simulink model "FixedWing_Dynamic_Model_SIL_simulink_PX4"  (R2023a)
settings: Solver=ode4  StartTime=0.0  StopTime=130  FixedStep=0.004  RelTol=1e-3
model workspace (MAT data in the model file):
  sample_time = 0.004
values from neighbouring files (symbols this model uses):
  env = struct    [InitEnvironment.m]
  frecuency = 0.012    [PX4_var_controllers.m]
  g = 9.81    [PX4_var_controllers.m]
  home_alt = 171    [InitSimulinkPlantVars.m]    (also in PX4_var_controllers.m)
  home_lat = 39.49738807491014    (= 39.4973880749)    [InitSimulinkPlantVars.m]    (also in PX4_var_controllers.m)
  home_lon = -0.6268122488722822    (= -0.626812248872)    [InitSimulinkPlantVars.m]    (also in PX4_var_controllers.m)
  mission = [wp]    [PX4_var_controllers.m]
  nwap = 9    [PX4_var_controllers.m]
  pitch_D = 0    [PX4_var_controllers.m]
  pitch_ff = 0.4    [PX4_var_controllers.m]
  pitch_I = 0.05    [PX4_var_controllers.m]
  pitch_P = 0.05    [PX4_var_controllers.m]
  poswp = [poswp1;poswp2;poswp3;poswp4;poswp5;poswp6;poswp7;poswp8;poswp9]    [PX4_var_controllers.m]
  roll_D = 0    [PX4_var_controllers.m]
  roll_ff = 0.4    [PX4_var_controllers.m]
  roll_I = 0.13    [PX4_var_controllers.m]
  roll_P = 0.085    [PX4_var_controllers.m]
  tc_pitch = 0.4    [PX4_var_controllers.m]
  tc_roll = 0.45    [PX4_var_controllers.m]
  uavData = struct    [InitFixedWingParam.m]
  V_cruise = [15,15,15,20,25,25,20,15,15]    [PX4_var_controllers.m]
  yaw_D = 0    [PX4_var_controllers.m]
  yaw_ff = 0.3    [PX4_var_controllers.m]
  yaw_I = 0.1    [PX4_var_controllers.m]
  yaw_P = 0.05    [PX4_var_controllers.m]
undefined symbols (not defined in the file or in its folder): DiscIntNeverNeededParam, Earth, LC, TEBCL, TECL, TECS, WGS84
libraries: aerolibactuator x5, aerolibasang x4, slpidlib x3, uavalgslib x2, aerolibatmos2 x2, shared6dof x1, aerolibtransform2 x1, aerolibconvert2 x1, simulink_extras x1
(part 2 of 3)

== system FixedWing_Dynamic_Model_SIL_simulink_PX4/Dynamics/Fixed-wing UAV Dynamics/Force and Moment Calculation ==
  note: M. Lizarraga. Design, Implementation and Flight Verification of a Versatile and Rapidly Reconfigurable UAV GNC Research Platform. PhD Dissertation, UC, Santa Cruz, Santa Cruz, CA, USA, 2009
  DCMbe : Inport
  Ve : Inport  Port=2
  Xe : Inport  Port=3
  pqr_b : Inport  Port=4
  rpy : Inport  Port=5
  Inputs : Inport  Port=6
  Actuator Model : Subsystem
  Add : Sum  Inputs=4
  Add1 : Sum  Inputs=2
  Aerodynamic Forces and Moments : Subsystem
  Bus Selector : BusSelector  OutputSignals=airspeed
  Constant : Constant  Value=[0 0 0]
  Gravity : Subsystem
  Ground Model : Subsystem
  Motor Model : Subsystem
  Terminator : Terminator
  F_xyz : Outport
  M_xyz : Outport  Port=2
  Airspeed : Outport  Port=3
  wires:
  Add/1 -> F_xyz/1
  DCMbe/1 -> Aerodynamic Forces and Moments/4(DCM_be), Ground Model/1(DCMbe), Gravity/1(DCM_be)
  pqr_b/1 -> Ground Model/5(pqr_b), Aerodynamic Forces and Moments/6(pqr_b)
  Actuator Model/1(ctrlSurfaces) -> Aerodynamic Forces and Moments/1(CtrlSurfaces), Motor Model/1(Ctrl Surfaces)
  Aerodynamic Forces and Moments/1(AirData) -> Bus Selector/1, Motor Model/2(Air Data)
  Ground Model/1(Fb_contact) -> Add/4
  Gravity/1(Fb_g) -> Add/3
  Motor Model/1(Fb_motor) -> Add/1
  Ve/1 -> Aerodynamic Forces and Moments/3(Ve), Ground Model/3(Ve)
  Ground Model/3(Crash_flag) -> Terminator/1
  Aerodynamic Forces and Moments/2(Fb_aero) -> Add/2
  Aerodynamic Forces and Moments/3(Mb_aero) -> Add1/1
  Xe/1 -> Aerodynamic Forces and Moments/5(Xe), Ground Model/2(Xe)
  Constant/1 -> Aerodynamic Forces and Moments/2(Wind_e)
  Inputs/1 -> Actuator Model/1(CtrlCmds)
  Bus Selector/1 -> Airspeed/1  "<airspeed>"
  rpy/1 -> Ground Model/4(rpy)
  Add1/1 -> M_xyz/1
  Ground Model/2(Mb_contact) -> Add1/2

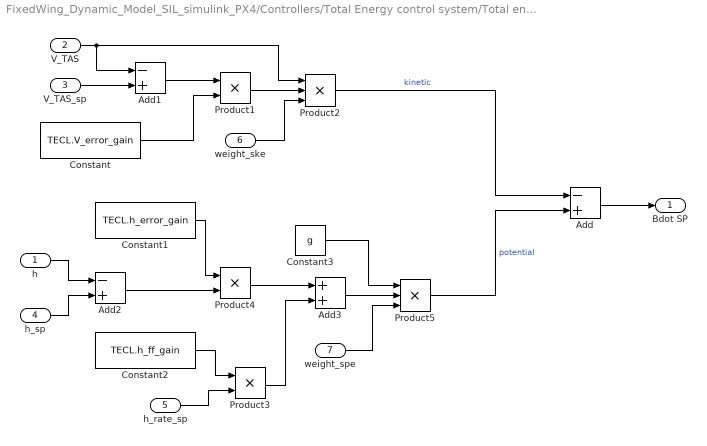
== system FixedWing_Dynamic_Model_SIL_simulink_PX4/Controllers/Total Energy control system/Total energy balance control loop/ B SP dot ==
  h : Inport  SampleTime=frecuency
  V_TAS : Inport  Port=2  SampleTime=frecuency
  V_TAS_sp : Inport  Port=3  SampleTime=frecuency
  h_sp : Inport  Port=4  SampleTime=frecuency
  h_rate_sp : Inport  Port=5  SampleTime=frecuency
  weight_ske : Inport  Port=6  SampleTime=frecuency
  weight_spe : Inport  Port=7  SampleTime=frecuency
  Add : Sum  Inputs=-+
  Add1 : Sum  Inputs=-+
  Add2 : Sum  Inputs=-+
  Add3 : Sum
  Constant : Constant  Value=TECL.V_error_gain  SampleTime=frecuency
  Constant1 : Constant  Value=TECL.h_error_gain  SampleTime=frecuency
  Constant2 : Constant  Value=TECL.h_ff_gain  SampleTime=frecuency
  Constant3 : Constant  Value=g  SampleTime=frecuency
  Product1 : Product
  Product2 : Product  Inputs=3
  Product3 : Product
  Product4 : Product
  Product5 : Product  Inputs=3
  Bdot SP : Outport  SampleTime=frecuency
  wires:
  V_TAS_sp/1 -> Add1/2
  Product1/1 -> Product2/2
  Product2/1 -> Add/1  "kinetic"
  h_sp/1 -> Add2/2
  h/1 -> Add2/1
  Add2/1 -> Product4/2
  Constant1/1 -> Product4/1
  Product4/1 -> Add3/1
  Constant2/1 -> Product3/1
  Product3/1 -> Add3/2
  Add3/1 -> Product5/2
  Constant3/1 -> Product5/1
  Product5/1 -> Add/2  "potential"
  Add/1 -> Bdot SP/1
  h_rate_sp/1 -> Product3/2
  weight_ske/1 -> Product2/3
  weight_spe/1 -> Product5/3
  V_TAS/1 -> Add1/1, Product2/1
  Add1/1 -> Product1/1
  Constant/1 -> Product1/2

== system FixedWing_Dynamic_Model_SIL_simulink_PX4/Controllers/Total Energy control system/Total energy balance control loop/Bdot ==
  V_TAS : Inport  SampleTime=frecuency
  V_rate : Inport  Port=2  SampleTime=frecuency
  h_rate : Inport  Port=3  SampleTime=frecuency
  weight_ske : Inport  Port=4  SampleTime=frecuency
  weight_spe : Inport  Port=5  SampleTime=frecuency
  Add : Sum  Inputs=-+
  Constant : Constant  Value=g  SampleTime=frecuency
  Product : Product  Inputs=3
  Product1 : Product  Inputs=3
  Bdot : Outport  SampleTime=frecuency
  wires:
  V_rate/1 -> Product/2
  Constant/1 -> Product1/3
  h_rate/1 -> Product1/2
  Product/1 -> Add/1  "kinetic"
  Product1/1 -> Add/2  "potential"
  Add/1 -> Bdot/1
  weight_ske/1 -> Product/3
  weight_spe/1 -> Product1/1
  V_TAS/1 -> Product/1

== system FixedWing_Dynamic_Model_SIL_simulink_PX4/Controllers/Total Energy control system/Total energy balance control loop/pitchdotsp - pitchFF ==
  Bdot SP : Inport  SampleTime=frecuency
  Gain : Gain  Gain=TEBCL.rate_ff
  pitch_FF : Outport  SampleTime=frecuency
  wires:
  Bdot SP/1 -> Gain/1
  Gain/1 -> pitch_FF/1

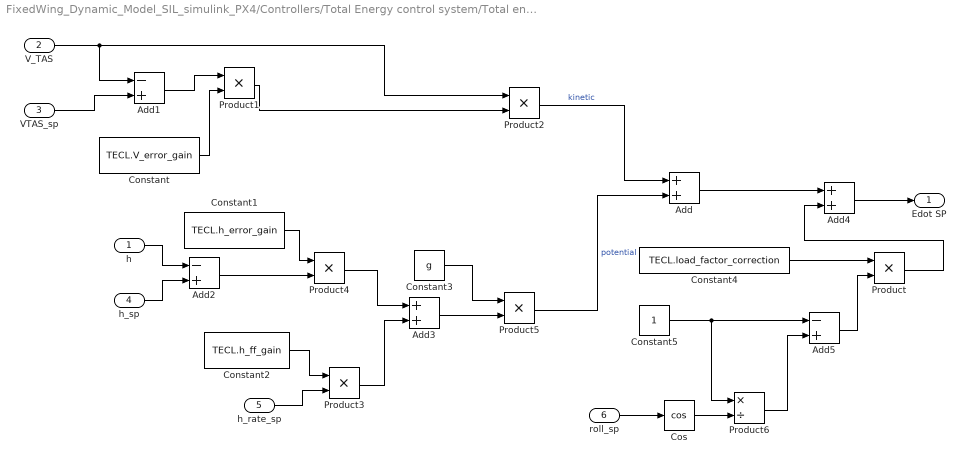
== system FixedWing_Dynamic_Model_SIL_simulink_PX4/Controllers/Total Energy control system/Total energy control loop/E SP dot ==
  h : Inport  SampleTime=frecuency
  V_TAS : Inport  Port=2  SampleTime=frecuency
  VTAS_sp : Inport  Port=3  SampleTime=frecuency
  h_sp : Inport  Port=4  SampleTime=frecuency
  h_rate_sp : Inport  Port=5  SampleTime=frecuency
  roll_sp : Inport  Port=6  SampleTime=frecuency
  Add : Sum
  Add1 : Sum  Inputs=-+
  Add2 : Sum  Inputs=-+
  Add3 : Sum
  Add4 : Sum
  Add5 : Sum  Inputs=-+
  Constant : Constant  Value=TECL.V_error_gain  SampleTime=frecuency
  Constant1 : Constant  Value=TECL.h_error_gain  SampleTime=frecuency
  Constant2 : Constant  Value=TECL.h_ff_gain  SampleTime=frecuency
  Constant3 : Constant  Value=g
  Constant4 : Constant  Value=TECL.load_factor_correction  SampleTime=frecuency
  Constant5 : Constant
  Cos : Trigonometry  Operator=cos
  Product{,1..5} (6 alike) : Product
  Product6 : Product  Inputs=*/
  Edot SP : Outport  SampleTime=frecuency
  wires:
  VTAS_sp/1 -> Add1/2
  Product2/1 -> Add/1  "kinetic"
  h_sp/1 -> Add2/2
  h/1 -> Add2/1
  Add2/1 -> Product4/2
  Constant1/1 -> Product4/1
  Product4/1 -> Add3/1
  Constant2/1 -> Product3/1
  Product3/1 -> Add3/2
  Add3/1 -> Product5/2
  Constant3/1 -> Product5/1
  Product5/1 -> Add/2  "potential"
  h_rate_sp/1 -> Product3/2
  Add/1 -> Add4/1
  Add4/1 -> Edot SP/1
  Constant4/1 -> Product/1
  Product/1 -> Add4/2
  Constant5/1 -> Add5/1, Product6/1
  Add5/1 -> Product/2
  roll_sp/1 -> Cos/1
  Cos/1 -> Product6/2
  Product6/1 -> Add5/2
  Constant/1 -> Product1/2
  Add1/1 -> Product1/1
  Product1/1 -> Product2/2
  V_TAS/1 -> Product2/1, Add1/1

== system FixedWing_Dynamic_Model_SIL_simulink_PX4/Controllers/Total Energy control system/Total energy control loop/Edot ==
  V_TAS : Inport  SampleTime=frecuency
  V_rate : Inport  Port=2  SampleTime=frecuency
  h_rate : Inport  Port=3  SampleTime=frecuency
  Add : Sum
  Constant : Constant  Value=g  SampleTime=frecuency
  Product : Product
  Product1 : Product
  Edot : Outport  SampleTime=frecuency
  wires:
  V_TAS/1 -> Product/1
  V_rate/1 -> Product/2
  Constant/1 -> Product1/2
  h_rate/1 -> Product1/1
  Product/1 -> Add/1  "kinetic"
  Product1/1 -> Add/2  "potential"
  Add/1 -> Edot/1

== system FixedWing_Dynamic_Model_SIL_simulink_PX4/Controllers/Total Energy control system/Total energy control loop/Subsystem ==
  ratio_undersped : Inport  SampleTime=frecuency
  T_sp : Inport  Port=2  SampleTime=frecuency
  Tmax : Inport  Port=3  SampleTime=frecuency
  Add : Sum  Inputs=+-
  Add1 : Sum
  Constant : Constant  SampleTime=frecuency
  Product : Product
  Product1 : Product
  throttle_setpoint : Outport  SampleTime=frecuency
  wires:
  ratio_undersped/1 -> Product/1, Add/2
  Tmax/1 -> Product/2
  Constant/1 -> Add/1
  T_sp/1 -> Product1/1
  Add/1 -> Product1/2
  Product1/1 -> Add1/1
  Product/1 -> Add1/2
  Add1/1 -> throttle_setpoint/1

== system FixedWing_Dynamic_Model_SIL_simulink_PX4/Controllers/Total Energy control system/Total energy control loop/Subsystem1 ==
  throttle_integ_input : Inport  SampleTime=frecuency
  ste_rate_to_throttle : Inport  Port=2  SampleTime=frecuency
  ratio_undersped : Inport  Port=3  SampleTime=frecuency
  Add : Sum  Inputs=-+
  Constant : Constant  SampleTime=frecuency
  Product : Product  Inputs=3
  throttle_integ : Outport  SampleTime=frecuency
  wires:
  ratio_undersped/1 -> Add/1
  Constant/1 -> Add/2
  throttle_integ_input/1 -> Product/1
  ste_rate_to_throttle/1 -> Product/2
  Add/1 -> Product/3
  Product/1 -> throttle_integ/1

== system FixedWing_Dynamic_Model_SIL_simulink_PX4/Dynamics/Fixed-wing UAV Dynamics/Force and Moment Calculation/Actuator Model ==
  note: Simple Actuator Model
  note: MAIN1 : aileron
      | MAIN2 : elevator
      | MAIN3 : rudder
      | MAIN4 : throttle
  CtrlCmds : Inport
  Bus Creator1 : BusCreator  Inputs=5
  Constant : Constant  Value=0*pi/180
  Demux : Demux
  Linear Second Order Actuators : aerolibactuator/Linear Second-Order Actuator  wn_fin=35  z_fin=0.75  fin_act_0=0  fin_act_vel=0
      settings: AttributesFormatString=|
      | Nat Freq => %<wn_fin>
      | Damping => %<z_fin>
  Linear Second-Order Actuator{1..4} (4 alike) : aerolibactuator/Linear Second-Order Actuator  wn_fin=35  z_fin=0.75  fin_act_0=0  fin_act_vel=0
  Signal Specification{,1..3} (4 alike) : SignalSpecification  Unit=rad
  Signal Specification4 : SignalSpecification  Unit=%
  uavData.cntrl.aileronGain : Gain  Gain=uavData.cntrl.aieleronGain
  uavData.cntrl.elevatorGain : Gain  Gain=uavData.cntrl.elevatorGain
  uavData.cntrl.rudderGain : Gain  Gain=uavData.cntrl.rudderGain
  uavData.cntrl.throttleGain : Gain  Gain=uavData.cntrl.throttleGain
  ctrlSurfaces : Outport  VectorParamsAs1DForOutWhenUnconnected=off
  wires:
  uavData.cntrl.elevatorGain/1 -> Linear Second-Order Actuator4/1
  uavData.cntrl.aileronGain/1 -> Linear Second-Order Actuator3/1
  uavData.cntrl.rudderGain/1 -> Linear Second-Order Actuator2/1
  Constant/1 -> Linear Second-Order Actuator1/1
  Bus Creator1/1 -> ctrlSurfaces/1
  Linear Second-Order Actuator4/1 -> Signal Specification1/1  "dE"
  Linear Second-Order Actuator3/1 -> Signal Specification/1  "dA"
  Linear Second-Order Actuator2/1 -> Signal Specification2/1  "dR"
  Linear Second-Order Actuator1/1 -> Signal Specification3/1  "dF"
  CtrlCmds/1 -> Demux/1
  Signal Specification1/1 -> Bus Creator1/1
  Signal Specification/1 -> Bus Creator1/2
  Signal Specification2/1 -> Bus Creator1/3
  Signal Specification3/1 -> Bus Creator1/4
  Signal Specification4/1 -> Bus Creator1/5
  Demux/3 -> uavData.cntrl.rudderGain/1
  Demux/1 -> uavData.cntrl.elevatorGain/1
  Demux/2 -> uavData.cntrl.aileronGain/1
  Demux/4 -> uavData.cntrl.throttleGain/1
  uavData.cntrl.throttleGain/1 -> Linear Second Order Actuators/1
  Linear Second Order Actuators/1 -> Signal Specification4/1  "dT"

== system FixedWing_Dynamic_Model_SIL_simulink_PX4/Dynamics/Fixed-wing UAV Dynamics/Force and Moment Calculation/Aerodynamic Forces and Moments ==
  CtrlSurfaces : Inport
  Wind_e : Inport  Port=2
  Ve : Inport  Port=3
  DCM_be : Inport  Port=4
  Xe : Inport  Port=5
  pqr_b : Inport  Port=6
  Compute Air Data : Subsystem  TreatAsAtomicUnit=on  VariantControl=use_aerospace_blocks == 1
  Compute Body Frame Forces and Moments : Subsystem
  Compute Rho : Subsystem
  Rotate Vw : Subsystem
  Vair : Sum  Inputs=+-  InputSameDT=on  SaturateOnIntegerOverflow=on  OutDataTypeStr=Inherit: Same as first input
  AirData : Outport  VectorParamsAs1DForOutWhenUnconnected=off
  Fb_aero : Outport  Port=2
  Mb_aero : Outport  Port=3
  wires:
  Ve/1 -> Vair/1
  Compute Body Frame Forces and Moments/1(F_b) -> Fb_aero/1
  Wind_e/1 -> Vair/2
  CtrlSurfaces/1 -> Compute Body Frame Forces and Moments/2(CtrlSurfaces)
  Compute Air Data/1(AirData) -> Compute Body Frame Forces and Moments/1(AirData), AirData/1
  Compute Body Frame Forces and Moments/2(M_b) -> Mb_aero/1
  Rotate Vw/1(Vb) -> Compute Air Data/1(Vb)
  Compute Rho/1(Rho) -> Compute Air Data/2(Rho)
  Vair/1 -> Rotate Vw/1(Vw)
  pqr_b/1 -> Compute Body Frame Forces and Moments/3(p,q,r)
  DCM_be/1 -> Rotate Vw/2(DCM_be)
  Xe/1 -> Compute Rho/1(Xe)

== system FixedWing_Dynamic_Model_SIL_simulink_PX4/Dynamics/Fixed-wing UAV Dynamics/Force and Moment Calculation/Gravity ==
  DCM_be : Inport
  Constant : Constant  Value=[0 0 env.ISA_g]'
  Gain : Gain  Gain=uavData.geometry.mass
  Matrix Multiply : Product  Multiplication=Matrix(*)
  Fb_g : Outport
  wires:
  Matrix Multiply/1 -> Gain/1
  Constant/1 -> Matrix Multiply/2
  DCM_be/1 -> Matrix Multiply/1
  Gain/1 -> Fb_g/1

== system FixedWing_Dynamic_Model_SIL_simulink_PX4/Dynamics/Fixed-wing UAV Dynamics/Force and Moment Calculation/Ground Model ==
  note: Body is assumed to be a rigid point mass on ground for contact force calculations.
      |
      | Normal force is modelled as a spring mass damper.
      |
      | Friction is modelled using Soft Coulomb model.
  DCMbe : Inport
  Xe : Inport  Port=2
  Ve : Inport  Port=3
  rpy : Inport  Port=4
  pqr_b : Inport  Port=5
  Constant : Constant  Value=[0 0 0]
  Crash Detector : Subsystem
  Friction Force : Subsystem
  Matrix Multiply : Product  Multiplication=Matrix(*)
  Mux1 : Mux  Inputs=2
  Normal Force : Subsystem
  Selector : Selector  InputPortWidth=3  IndexOptions=Index vector (dialog)  Indices=[3]  OutputSizes=1
  Selector1 : Selector  InputPortWidth=3  IndexOptions=Index vector (dialog)  Indices=[3]  OutputSizes=1
  Selector2 : Selector  InputPortWidth=3  IndexOptions=Index vector (dialog)  Indices=[1,2]  OutputSizes=1
  Terminator : Terminator
  Terminator1 : Terminator
  Unary Minus1 : UnaryMinus
  Fb_contact : Outport
  Mb_contact : Outport  Port=2
  Crash_flag : Outport  Port=3
  wires:
  Crash Detector/1(crashFlag) -> Crash_flag/1
  Xe/1 -> Selector/1
  Ve/1 -> Selector2/1, Selector1/1
  Selector1/1 -> Normal Force/1(Vz)
  Selector/1 -> Normal Force/2(Z)
  DCMbe/1 -> Matrix Multiply/1
  Matrix Multiply/1 -> Fb_contact/1
  Normal Force/1(Normal) -> Friction Force/2(Fn), Unary Minus1/1
  Mux1/1 -> Matrix Multiply/2, Crash Detector/1(F)
  Unary Minus1/1 -> Mux1/2
  Selector2/1 -> Friction Force/1(V)
  Friction Force/1(Friction) -> Mux1/1
  pqr_b/1 -> Terminator/1
  rpy/1 -> Terminator1/1
  Constant/1 -> Mb_contact/1

== system FixedWing_Dynamic_Model_SIL_simulink_PX4/Dynamics/Fixed-wing UAV Dynamics/Force and Moment Calculation/Motor Model ==
  Ctrl Surfaces : Inport
  Air Data : Inport  Port=2
  Bus Selector : BusSelector  OutputSignals=dT
  Bus Selector1 : BusSelector  OutputSignals=airspeed
  Engine Model : Subsystem
  Fb_motor : Outport  VectorParamsAs1DForOutWhenUnconnected=off
  wires:
  Bus Selector1/1 -> Engine Model/2(Airspeed)  "<airspeed>"
  Ctrl Surfaces/1 -> Bus Selector/1
  Air Data/1 -> Bus Selector1/1
  Bus Selector/1 -> Engine Model/1(dt)  "<dT>"
  Engine Model/1(Thrust_b) -> Fb_motor/1

== system FixedWing_Dynamic_Model_SIL_simulink_PX4/Dynamics/Fixed-wing UAV Dynamics/Force and Moment Calculation/Aerodynamic Forces and Moments/Compute Air Data ==
  Vb : Inport  PortDimensions=3
  Rho : Inport  Port=2
  Bus Creator : BusCreator  Inputs=4
  Demux : Demux  Outputs=3
  Dynamic Pressure : aerolibasang/Dynamic Pressure
  Subsystem : Subsystem
  AirData : Outport  VectorParamsAs1DForOutWhenUnconnected=off
  wires:
  Bus Creator/1 -> AirData/1
  Rho/1 -> Dynamic Pressure/2
  Dynamic Pressure/1 -> Bus Creator/4  "q"
  Vb/1 -> Subsystem/1(Vb), Dynamic Pressure/1
  Subsystem/1(airData) -> Demux/1
  Demux/1 -> Bus Creator/1  "alpha"
  Demux/2 -> Bus Creator/2  "beta"
  Demux/3 -> Bus Creator/3  "airspeed"

== system FixedWing_Dynamic_Model_SIL_simulink_PX4/Dynamics/Fixed-wing UAV Dynamics/Force and Moment Calculation/Aerodynamic Forces and Moments/Compute Body Frame Forces and Moments ==
  AirData : Inport
  CtrlSurfaces : Inport  Port=2
  p,q,r : Inport  Port=3
  Bus Selector : BusSelector  OutputSignals=alpha,beta
  Mux : Mux  Inputs=2
  Rotate FM to body frame : Subsystem
  Wind frame F& M : Subsystem
  F_b : Outport  Unit=kg*m/s^2  VectorParamsAs1DForOutWhenUnconnected=off
  M_b : Outport  Port=2  Unit=N*m  VectorParamsAs1DForOutWhenUnconnected=off
  wires:
  Mux/1 -> Rotate FM to body frame/2(alpha_beta)
  Bus Selector/2 -> Mux/2  "<beta>"
  Bus Selector/1 -> Mux/1  "<alpha>"
  Wind frame F& M/1(FM_w) -> Rotate FM to body frame/1(FM_w)  "FM_W"
  p,q,r/1 -> Wind frame F& M/3(p,q,r)
  Rotate FM to body frame/2(M_b) -> M_b/1
  Rotate FM to body frame/1(F_b) -> F_b/1
  CtrlSurfaces/1 -> Wind frame F& M/2(CtrlSurfaces)
  AirData/1 -> Wind frame F& M/1(Airdata), Bus Selector/1

== system FixedWing_Dynamic_Model_SIL_simulink_PX4/Dynamics/Fixed-wing UAV Dynamics/Force and Moment Calculation/Aerodynamic Forces and Moments/Compute Rho ==
  Xe : Inport
  Gain : Gain  Gain=-1
      settings: AttributesFormatString=Z to Alt
  Get Z : Selector  InputPortWidth=3  IndexOptions=Index vector (dialog)  Indices=[3]  OutputSizes=[(-2)]
  ISA Atmosphere Model1 : aerolibatmos2/ISA Atmosphere Model  custom=on  g=env.ISA_g  gamma=1.4  R=env.ISA_R  L=env.ISA_lapse  h_trop=11000  h_strat=20000  rho0=env.ISA_rho0  P0=env.ISA_P0  T0=env.ISA_T0  h0=0
  Terminator : Terminator
  Terminator1 : Terminator
  Terminator2 : Terminator
  Transfer Fcn : TransferFcn  Denominator=[.01 1]
  Rho : Outport  VectorParamsAs1DForOutWhenUnconnected=off
  wires:
  ISA Atmosphere Model1/2 -> Terminator1/1
  ISA Atmosphere Model1/1 -> Terminator/1  "OAT"
  Gain/1 -> ISA Atmosphere Model1/1
  Get Z/1 -> Transfer Fcn/1
  Transfer Fcn/1 -> Gain/1
  ISA Atmosphere Model1/3 -> Terminator2/1  "static"
  Xe/1 -> Get Z/1
  ISA Atmosphere Model1/4 -> Rho/1

== system FixedWing_Dynamic_Model_SIL_simulink_PX4/Dynamics/Fixed-wing UAV Dynamics/Force and Moment Calculation/Aerodynamic Forces and Moments/Rotate Vw ==
  Vw : Inport
  DCM_be : Inport  Port=2
  RL2B * Vw : Product  Multiplication=Matrix(*)  InputSameDT=on  SaturateOnIntegerOverflow=on  OutDataTypeStr=Inherit: Same as first input
  Vb : Outport  Unit=m/s  VectorParamsAs1DForOutWhenUnconnected=off
  wires:
  RL2B * Vw/1 -> Vb/1
  Vw/1 -> RL2B * Vw/2
  DCM_be/1 -> RL2B * Vw/1

== system FixedWing_Dynamic_Model_SIL_simulink_PX4/Dynamics/Fixed-wing UAV Dynamics/Force and Moment Calculation/Ground Model/Crash Detector ==
  F : Inport
  Constant : Constant  Value=true
  Constant1 : Constant  Value=false
  Gain : Gain  Gain=1/(env.ISA_g*uavData.geometry.mass)
  Switch : Switch  Criteria=u2 > Threshold  Threshold=uavData.contact.gLimit  SaturateOnIntegerOverflow=off  InputSameDT=off
  norm1 : Subsystem
  crashFlag : Outport
  wires:
  F/1 -> norm1/1(F)
  norm1/1(Out1) -> Gain/1
  Switch/1 -> crashFlag/1
  Constant/1 -> Switch/1
  Constant1/1 -> Switch/3
  Gain/1 -> Switch/2

== system FixedWing_Dynamic_Model_SIL_simulink_PX4/Dynamics/Fixed-wing UAV Dynamics/Force and Moment Calculation/Ground Model/Friction Force ==
  V : Inport
  Fn : Inport  Port=2
  Product : Product
  Soft Coulomb Friction : Subsystem
  Unary Minus : UnaryMinus
  Friction : Outport
  wires:
  Fn/1 -> Product/2
  Soft Coulomb Friction/1(Out1) -> Product/1
  Product/1 -> Unary Minus/1
  Unary Minus/1 -> Friction/1
  V/1 -> Soft Coulomb Friction/1(V)

== system FixedWing_Dynamic_Model_SIL_simulink_PX4/Dynamics/Fixed-wing UAV Dynamics/Force and Moment Calculation/Ground Model/Normal Force ==
  Vz : Inport
  Z : Inport  Port=2
  Add : Sum
  Constant : Constant  Value=0
  Damper : Gain  Gain=-uavData.contact.damper
  Saturation : Saturate  UpperLimit=inf  LowerLimit=0
  Spring Kp : Gain  Gain=-uavData.contact.spring
  Switch : Switch  Criteria=u2 > Threshold  SaturateOnIntegerOverflow=off  InputSameDT=off
  Unary Minus : UnaryMinus
  Unary Minus1 : UnaryMinus
  Normal : Outport
  wires:
  Constant/1 -> Switch/1
  Z/1 -> Unary Minus/1
  Switch/1 -> Saturation/1
  Damper/1 -> Add/2
  Add/1 -> Switch/3
  Spring Kp/1 -> Add/1
  Vz/1 -> Unary Minus1/1
  Saturation/1 -> Normal/1
  Unary Minus/1 -> Spring Kp/1, Switch/2
  Unary Minus1/1 -> Damper/1

== system FixedWing_Dynamic_Model_SIL_simulink_PX4/Dynamics/Fixed-wing UAV Dynamics/Force and Moment Calculation/Motor Model/Engine Model ==
  dt : Inport
  Airspeed : Inport  Port=2
  Constant4 : Constant  Value=0
      settings: AttributesFormatString=%<Value>
  Get To : Subsystem
  Mass Conversion : aerolibconvert2/Mass Conversion  IU=lbm  OU=kg
  Mux : Mux  Inputs=2
  Mux1 : Mux  Inputs=3
  Saturation : Saturate  UpperLimit=inf  LowerLimit=0
  Thrust Available (lbs) : Fcn  Expr=u(1) - 0.047*sqrt(u(1))*u(2)
  kg2N : Gain  Gain=env.ISA_g  SaturateOnIntegerOverflow=on  OutDataTypeStr=Inherit: Same as input  ParamDataTypeStr=Inherit: Same as input
      settings: AttributesFormatString=%<Gain>
  Thrust_b : Outport  Unit=kg*m/s^2  VectorParamsAs1DForOutWhenUnconnected=off
  wires:
  Constant4/1 -> Mux1/3, Mux1/2
  Mass Conversion/1 -> kg2N/1
  Mux1/1 -> Thrust_b/1
  Airspeed/1 -> Mux/2
  Thrust Available (lbs)/1 -> Mass Conversion/1
  Mux/1 -> Thrust Available (lbs)/1
  Get To/1(To) -> Mux/1
  dt/1 -> Get To/1(dt)
  kg2N/1 -> Saturation/1
  Saturation/1 -> Mux1/1

== system FixedWing_Dynamic_Model_SIL_simulink_PX4/Dynamics/Fixed-wing UAV Dynamics/Force and Moment Calculation/Aerodynamic Forces and Moments/Compute Air Data/Subsystem ==
  note: Avoid singularity at low speeds
  Vb : Inport
  "Incidence, Sideslip, & Airspeed" : aerolibasang/Incidence, Sideslip, & Airspeed
  Mux : Mux  Inputs=3
  Mux1 : Mux  Inputs=3
  Switch : Switch  Criteria=u2 > Threshold  Threshold=0.1  SaturateOnIntegerOverflow=off  InputSameDT=off
  alpha : Constant  Value=0
  beta : Constant  Value=0
  norm : Subsystem
  airData : Outport
  wires:
  "Incidence, Sideslip, & Airspeed"/1 -> Mux/1  "alpha"
  "Incidence, Sideslip, & Airspeed"/3 -> Mux/3  "airspeed"
  Vb/1 -> norm/1(In1), "Incidence, Sideslip, & Airspeed"/1
  norm/1(Out1) -> Mux1/3, Switch/2
  "Incidence, Sideslip, & Airspeed"/2 -> Mux/2  "beta"
  Switch/1 -> airData/1
  Mux/1 -> Switch/1
  alpha/1 -> Mux1/1
  beta/1 -> Mux1/2
  Mux1/1 -> Switch/3

== system FixedWing_Dynamic_Model_SIL_simulink_PX4/Dynamics/Fixed-wing UAV Dynamics/Force and Moment Calculation/Aerodynamic Forces and Moments/Compute Body Frame Forces and Moments/Rotate FM to body frame ==
  FM_w : Inport
  alpha_beta : Inport  Port=2
  Forces : Selector  InputPortWidth=6  IndexOptions=Index vector (dialog)  Indices=[1 2 3]  OutputSizes=[(-2)]
  Moments : Selector  InputPortWidth=6  IndexOptions=Index vector (dialog)  Indices=[4 5 6]  OutputSizes=[(-2)]
  Rotate Forces : Subsystem
  Rotate Moments : Subsystem
  F_b : Outport  VectorParamsAs1DForOutWhenUnconnected=off
  M_b : Outport  Port=2  VectorParamsAs1DForOutWhenUnconnected=off
  wires:
  alpha_beta/1 -> Rotate Forces/2(alpha_beta), Rotate Moments/1(alpha_beta)
  Moments/1 -> Rotate Moments/2(M_w)
  FM_w/1 -> Forces/1, Moments/1
  Forces/1 -> Rotate Forces/1(F_w)
  Rotate Moments/1(M_b) -> M_b/1
  Rotate Forces/1(F_b) -> F_b/1

== system FixedWing_Dynamic_Model_SIL_simulink_PX4/Dynamics/Fixed-wing UAV Dynamics/Force and Moment Calculation/Aerodynamic Forces and Moments/Compute Body Frame Forces and Moments/Wind frame F& M ==
  Airdata : Inport
  CtrlSurfaces : Inport  Port=2
  p,q,r : Inport  Port=3
  Bus Creator1 : BusCreator  Inputs=2
  Bus Selector1 : BusSelector  OutputSignals=dA,dR
  Bus Selector2 : BusSelector  OutputSignals=dE,dF
  Bus Selector6 : BusSelector  OutputSignals=beta,airspeed
  Bus Selector7 : BusSelector  OutputSignals=alpha,airspeed
  Get Forces and Moments : Subsystem
  Lateral Channel : Subsystem
  Longitudinal Channel : Subsystem
  FM_w : Outport  PortDimensions=6  VectorParamsAs1DForOutWhenUnconnected=off
  wires:
  Get Forces and Moments/1(FM_w) -> FM_w/1
  Bus Creator1/1 -> Get Forces and Moments/2(AeroCoeffs)
  Bus Selector7/2 -> Longitudinal Channel/2(Airpseed)  "<airspeed>"
  Bus Selector7/1 -> Longitudinal Channel/1(alpha)  "<alpha>"
  Bus Selector6/2 -> Lateral Channel/2(Airspeed)  "<airspeed>"
  Bus Selector6/1 -> Lateral Channel/1(beta)  "<beta>"
  Airdata/1 -> Bus Selector6/1, Bus Selector7/1, Get Forces and Moments/1(Airdata)
  Bus Selector2/2 -> Longitudinal Channel/4(dF)  "<dF>"
  Bus Selector2/1 -> Longitudinal Channel/3(dE)  "<dE>"
  Bus Selector1/2 -> Lateral Channel/4(dR)  "<dR>"
  Bus Selector1/1 -> Lateral Channel/3(dA)  "<dA>"
  CtrlSurfaces/1 -> Bus Selector1/1, Bus Selector2/1
  p,q,r/1 -> Lateral Channel/5(p,q,r), Longitudinal Channel/5(p,q,r)
  Lateral Channel/1(Lateral) -> Bus Creator1/1
  Longitudinal Channel/1(Longitudinal) -> Bus Creator1/2

== system FixedWing_Dynamic_Model_SIL_simulink_PX4/Dynamics/Fixed-wing UAV Dynamics/Force and Moment Calculation/Ground Model/Crash Detector/norm1 ==
  F : Inport
  Dot Product : DotProduct  OutDataTypeStr=Inherit: Inherit via internal rule
  Sqrt : Sqrt
  Out1 : Outport
  wires:
  Dot Product/1 -> Sqrt/1
  F/1 -> Dot Product/2, Dot Product/1
  Sqrt/1 -> Out1/1

== system FixedWing_Dynamic_Model_SIL_simulink_PX4/Dynamics/Fixed-wing UAV Dynamics/Force and Moment Calculation/Ground Model/Friction Force/Soft Coulomb Friction ==
  note: Pennestrì, E., Rossi, V., Salvini, P. et al. Review and comparison of dry friction force models. Nonlinear Dyn 83, 1785–1801 (2016). https://doi.org/10.1007/s11071-015-2485-3
  V : Inport
  Tanh : Trigonometry  Operator=tanh
  friction coefficient : Gain  Gain=uavData.contact.rollingFriction
  vd : Gain  Gain=1/uavData.contact.vd
  Out1 : Outport
  wires:
  V/1 -> vd/1
  vd/1 -> Tanh/1
  Tanh/1 -> friction coefficient/1
  friction coefficient/1 -> Out1/1

== system FixedWing_Dynamic_Model_SIL_simulink_PX4/Dynamics/Fixed-wing UAV Dynamics/Force and Moment Calculation/Motor Model/Engine Model/Get To ==
  dt : Inport
  Divide : Product  Inputs=3
  Math Function : Math  Operator=pow  SignedPower=on
  Math Function1 : Math  Operator=pow  SignedPower=on
  MaxRPM : Gain  Gain=7200  SaturateOnIntegerOverflow=on  OutDataTypeStr=Inherit: Same as input  ParamDataTypeStr=Inherit: Same as input
      settings: AttributesFormatString=%<Gain>
  MaxRPM1 : Gain  Gain=uavData.engine.TFact  SaturateOnIntegerOverflow=on  OutDataTypeStr=Inherit: Same as input  ParamDataTypeStr=Inherit: Same as input
      settings: AttributesFormatString=%<Gain>
  Min RPM : Constant  Value=2000
      settings: AttributesFormatString=%<Value>
  Min Th K : Constant  Value=uavData.engine.MinThK
      settings: AttributesFormatString=%<Value>
  Prop Diameter (in) : Constant  Value=17
      settings: AttributesFormatString=%<Value>
  Prop Diameter (in)1 : Constant  Value=2
      settings: AttributesFormatString=%<Value>
  Prop Diameter (in)2 : Constant  Value=4
      settings: AttributesFormatString=%<Value>
  Saturation : Saturate  UpperLimit=1.0  LowerLimit=0
      settings: AttributesFormatString="[%<LowerLimit>  %<UpperLimit>]"
  Sum : Sum  Inputs=|++
  Sum1 : Sum  Inputs=|++
  Th K : Gain  Gain=uavData.engine.ThK  SaturateOnIntegerOverflow=on  OutDataTypeStr=Inherit: Same as input  ParamDataTypeStr=Inherit: Same as input
      settings: AttributesFormatString=%<Gain>
  To Constant : Constant  Value=2.83e-12
      settings: AttributesFormatString=%<Value>
  To : Outport  VectorParamsAs1DForOutWhenUnconnected=off
  wires:
  Min Th K/1 -> Sum1/2
  Sum1/1 -> MaxRPM/1
  dt/1 -> Saturation/1
  Th K/1 -> Sum1/1
  MaxRPM/1 -> Sum/1
  Min RPM/1 -> Sum/2
  Sum/1 -> Math Function/1
  MaxRPM1/1 -> To/1
  Divide/1 -> MaxRPM1/1
  To Constant/1 -> Divide/3
  Math Function1/1 -> Divide/2
  Math Function/1 -> Divide/1
  Prop Diameter (in)/1 -> Math Function1/1
  Prop Diameter (in)2/1 -> Math Function1/2
  Prop Diameter (in)1/1 -> Math Function/2
  Saturation/1 -> Th K/1

== system FixedWing_Dynamic_Model_SIL_simulink_PX4/Dynamics/Fixed-wing UAV Dynamics/Force and Moment Calculation/Aerodynamic Forces and Moments/Compute Air Data/Subsystem/norm ==
  In1 : Inport
  Dot Product : DotProduct  OutDataTypeStr=Inherit: Inherit via internal rule
  Sqrt : Sqrt
  Out1 : Outport
  wires:
  In1/1 -> Dot Product/2, Dot Product/1
  Dot Product/1 -> Sqrt/1
  Sqrt/1 -> Out1/1

== system FixedWing_Dynamic_Model_SIL_simulink_PX4/Dynamics/Fixed-wing UAV Dynamics/Force and Moment Calculation/Aerodynamic Forces and Moments/Compute Body Frame Forces and Moments/Rotate FM to body frame/Rotate Forces ==
  F_w : Inport
  alpha_beta : Inport  Port=2
  Product2 : Product  Multiplication=Matrix(*)  SaturateOnIntegerOverflow=on  OutDataTypeStr=Inherit: Same as first input
  RB2W : Subsystem
  RW2B : Math  Operator=transpose  SignedPower=on
  F_b : Outport  PortDimensions=3  VectorParamsAs1DForOutWhenUnconnected=off
  wires:
  RW2B/1 -> Product2/1
  F_w/1 -> Product2/2
  Product2/1 -> F_b/1
  alpha_beta/1 -> RB2W/1(aoa beta)
  RB2W/1(Rw2b) -> RW2B/1

== system FixedWing_Dynamic_Model_SIL_simulink_PX4/Dynamics/Fixed-wing UAV Dynamics/Force and Moment Calculation/Aerodynamic Forces and Moments/Compute Body Frame Forces and Moments/Rotate FM to body frame/Rotate Moments ==
  alpha_beta : Inport
  M_w : Inport  Port=2
  Matrix Multiply : Product  Multiplication=Matrix(*)
  RB2W : Subsystem
  RW2B : Math  Operator=transpose  SignedPower=on
  M_b : Outport  PortDimensions=3  VectorParamsAs1DForOutWhenUnconnected=off
  wires:
  RB2W/1(Rw2b) -> RW2B/1
  alpha_beta/1 -> RB2W/1(aoa beta)
  M_w/1 -> Matrix Multiply/2
  RW2B/1 -> Matrix Multiply/1
  Matrix Multiply/1 -> M_b/1

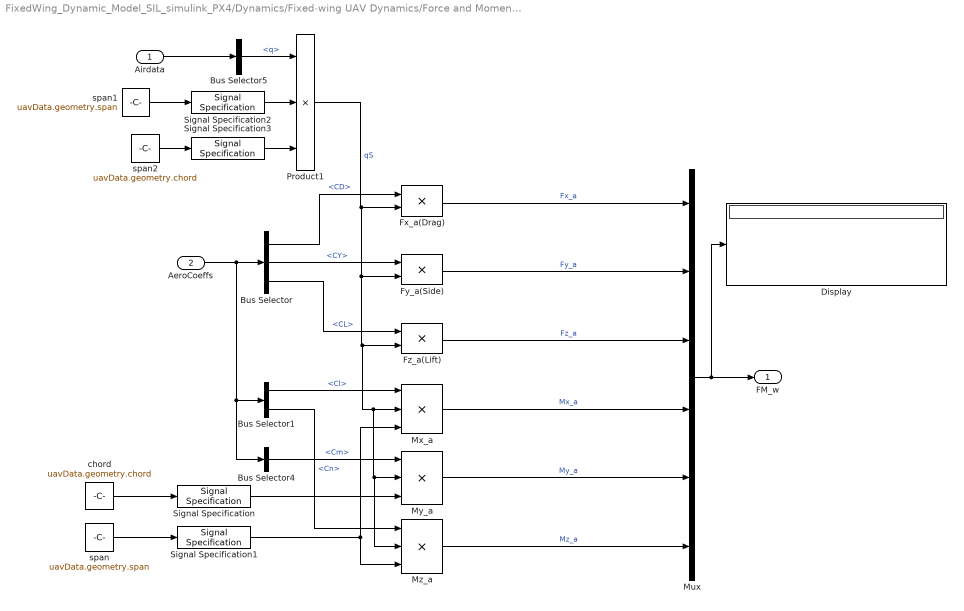
== system FixedWing_Dynamic_Model_SIL_simulink_PX4/Dynamics/Fixed-wing UAV Dynamics/Force and Moment Calculation/Aerodynamic Forces and Moments/Compute Body Frame Forces and Moments/Wind frame F& M/Get Forces and Moments ==
  Airdata : Inport
  AeroCoeffs : Inport  Port=2
  Bus Selector : BusSelector  OutputSignals=signal2.CD,signal1.CY,signal2.CL
  Bus Selector1 : BusSelector  OutputSignals=signal1.Cl,signal1.Cn
  Bus Selector4 : BusSelector  OutputSignals=signal2.Cm
  Bus Selector5 : BusSelector  OutputSignals=q
  Display : Display
  Fx_a(Drag) : Product  Inputs=**  SaturateOnIntegerOverflow=on  OutDataTypeStr=Inherit: Same as first input
  Fy_a(Side) : Product  SaturateOnIntegerOverflow=on  OutDataTypeStr=Inherit: Same as first input
  Fz_a(Lift) : Product  SaturateOnIntegerOverflow=on  OutDataTypeStr=Inherit: Same as first input
  Mux : Mux  Inputs=6
  Mx_a : Product  Inputs=3  SaturateOnIntegerOverflow=on  OutDataTypeStr=Inherit: Same as first input
  My_a : Product  Inputs=3  SaturateOnIntegerOverflow=on  OutDataTypeStr=Inherit: Same as first input
  Mz_a : Product  Inputs=3  SaturateOnIntegerOverflow=on  OutDataTypeStr=Inherit: Same as first input
  Product1 : Product  Inputs=3  SaturateOnIntegerOverflow=on  OutDataTypeStr=Inherit: Same as first input
  Signal Specification{,1..3} (4 alike) : SignalSpecification  Unit=m
  chord : Constant  Value=uavData.geometry.chord  VectorParams1D=off
      settings: AttributesFormatString=%<Value>
  span : Constant  Value=uavData.geometry.span  VectorParams1D=off
      settings: AttributesFormatString=%<Value>
  span1 : Constant  Value=uavData.geometry.span  VectorParams1D=off
      settings: AttributesFormatString=%<Value>
  span2 : Constant  Value=uavData.geometry.chord  VectorParams1D=off
      settings: AttributesFormatString=%<Value>
  FM_w : Outport  VectorParamsAs1DForOutWhenUnconnected=off
  wires:
  Mx_a/1 -> Mux/4  "Mx_a"
  Bus Selector/2 -> Fy_a(Side)/1  "<CY>"
  Bus Selector4/1 -> My_a/1  "<Cm>"
  span2/1 -> Signal Specification3/1
  Fx_a(Drag)/1 -> Mux/1  "Fx_a"
  Bus Selector/1 -> Fx_a(Drag)/1  "<CD>"
  AeroCoeffs/1 -> Bus Selector/1, Bus Selector1/1, Bus Selector4/1
  My_a/1 -> Mux/5  "My_a"
  Fz_a(Lift)/1 -> Mux/3  "Fz_a"
  Mz_a/1 -> Mux/6  "Mz_a"
  Airdata/1 -> Bus Selector5/1
  chord/1 -> Signal Specification/1
  span/1 -> Signal Specification1/1
  Fy_a(Side)/1 -> Mux/2  "Fy_a"
  Mux/1 -> FM_w/1, Display/1
  Bus Selector1/2 -> Mz_a/1  "<Cn>"
  Bus Selector/3 -> Fz_a(Lift)/1  "<CL>"
  Product1/1 -> Fx_a(Drag)/2, Fy_a(Side)/2, Fz_a(Lift)/2, Mx_a/2, My_a/2, Mz_a/2  "qS"
  span1/1 -> Signal Specification2/1
  Bus Selector1/1 -> Mx_a/1  "<Cl>"
  Bus Selector5/1 -> Product1/1  "<q>"
  Signal Specification/1 -> My_a/3
  Signal Specification1/1 -> Mz_a/3, Mx_a/3
  Signal Specification2/1 -> Product1/2
  Signal Specification3/1 -> Product1/3

== system FixedWing_Dynamic_Model_SIL_simulink_PX4/Dynamics/Fixed-wing UAV Dynamics/Force and Moment Calculation/Aerodynamic Forces and Moments/Compute Body Frame Forces and Moments/Wind frame F& M/Lateral Channel ==
  beta : Inport
  Airspeed : Inport  Port=2
  dA : Inport  Port=3
  dR : Inport  Port=4
  p,q,r : Inport  Port=5
  Bus Creator : BusCreator  Inputs=3
  CY : Subsystem
  Cl : Subsystem
  Cn : Subsystem
  Lateral : Outport  VectorParamsAs1DForOutWhenUnconnected=off
  wires:
  Cl/1(Cl) -> Bus Creator/2  "Cl"
  p,q,r/1 -> Cn/4(p,q,r), Cl/4(p,q,r)
  Airspeed/1 -> Cn/5(Airspeed), Cl/5(Airspeed)
  dR/1 -> CY/2(dR), Cl/3(dR), Cn/3(Dr)
  dA/1 -> Cl/2(dA), Cn/2(dA)
  beta/1 -> CY/1(beta), Cl/1(beta), Cn/1(beta)
  Cn/1(Cn) -> Bus Creator/3  "Cn"
  CY/1(CY) -> Bus Creator/1  "CY"
  Bus Creator/1 -> Lateral/1

== system FixedWing_Dynamic_Model_SIL_simulink_PX4/Dynamics/Fixed-wing UAV Dynamics/Force and Moment Calculation/Aerodynamic Forces and Moments/Compute Body Frame Forces and Moments/Wind frame F& M/Longitudinal Channel ==
  alpha : Inport
  Airpseed : Inport  Port=2
  dE : Inport  Port=3
  dF : Inport  Port=4
  p,q,r : Inport  Port=5
  Bus Creator : BusCreator  Inputs=3
  CD : Subsystem
  CL : Subsystem
  Cm : Subsystem
  Transfer Fcn : TransferFcn  Numerator=[1 0]  Denominator=[0.1 1]
  Y-down : Gain  Gain=-1  SaturateOnIntegerOverflow=on  OutDataTypeStr=Inherit: Same as input  ParamDataTypeStr=Inherit: Same as input
      settings: AttributesFormatString=%<Gain>
  Longitudinal : Outport  VectorParamsAs1DForOutWhenUnconnected=off
  wires:
  Transfer Fcn/1 -> CL/2(alpha_dot)
  Airpseed/1 -> CL/6(Airspeed)
  p,q,r/1 -> Cm/4(p,q,r), CL/5(p,q,r)
  dF/1 -> Cm/3(Df), CL/4(dF)
  Bus Creator/1 -> Longitudinal/1
  Cm/1(Cm) -> Bus Creator/3  "Cm"
  CL/1(CL) -> CD/1(CL), Y-down/1
  dE/1 -> Cm/2(De), CL/3(dE)
  Y-down/1 -> Bus Creator/2  "CL"
  CD/1(CD) -> Bus Creator/1  "CD"
  alpha/1 -> Transfer Fcn/1, Cm/1(alpha), CL/1(alpha)

== system FixedWing_Dynamic_Model_SIL_simulink_PX4/Dynamics/Fixed-wing UAV Dynamics/Force and Moment Calculation/Aerodynamic Forces and Moments/Compute Body Frame Forces and Moments/Rotate FM to body frame/Rotate Forces/RB2W ==
  aoa beta : Inport
  11 : Fcn  Expr=u[3]*u[4]
  12 : Fcn  Expr=u[2]
  13 : Fcn  Expr=u[1]*u[4]
  21 : Fcn  Expr=-u[3]*u[2]
  22 : Fcn  Expr=u[4]
  23 : Fcn  Expr=-u[1]*u[2]
  31 : Fcn  Expr=-u[1]
  32 : Fcn  Expr=0
  33 : Fcn  Expr=u[3]
  Mux : Mux  Inputs=2
  Mux3 : Mux  Inputs=9
  Reshape 9x1->3x3 : Reshape  OutputDimensionality=Customize  OutputDimensions=[3,3]
  sincos : Trigonometry  Operator=sincos
  Rw2b : Outport  VectorParamsAs1DForOutWhenUnconnected=off
  wires:
  Mux/1 -> 11/1, 21/1, 31/1, 12/1, 22/1, 32/1, 13/1, 23/1, 33/1
  aoa beta/1 -> sincos/1
  sincos/2 -> Mux/2
  sincos/1 -> Mux/1
  33/1 -> Mux3/9
  23/1 -> Mux3/8
  13/1 -> Mux3/7
  32/1 -> Mux3/6
  22/1 -> Mux3/5
  12/1 -> Mux3/4
  31/1 -> Mux3/3
  21/1 -> Mux3/2
  11/1 -> Mux3/1
  Reshape 9x1->3x3/1 -> Rw2b/1
  Mux3/1 -> Reshape 9x1->3x3/1

== system FixedWing_Dynamic_Model_SIL_simulink_PX4/Dynamics/Fixed-wing UAV Dynamics/Force and Moment Calculation/Aerodynamic Forces and Moments/Compute Body Frame Forces and Moments/Rotate FM to body frame/Rotate Moments/RB2W ==
  aoa beta : Inport
  11 : Fcn  Expr=u[3]*u[4]
  12 : Fcn  Expr=u[2]
  13 : Fcn  Expr=u[1]*u[4]
  21 : Fcn  Expr=-u[3]*u[2]
  22 : Fcn  Expr=u[4]
  23 : Fcn  Expr=-u[1]*u[2]
  31 : Fcn  Expr=-u[1]
  32 : Fcn  Expr=0
  33 : Fcn  Expr=u[3]
  Mux : Mux  Inputs=2
  Mux3 : Mux  Inputs=9
  Reshape 9x1->3x3 : Reshape  OutputDimensionality=Customize  OutputDimensions=[3,3]
  sincos : Trigonometry  Operator=sincos
  Rw2b : Outport  VectorParamsAs1DForOutWhenUnconnected=off
  wires:
  Mux/1 -> 11/1, 21/1, 31/1, 12/1, 22/1, 32/1, 13/1, 23/1, 33/1
  aoa beta/1 -> sincos/1
  sincos/2 -> Mux/2
  sincos/1 -> Mux/1
  33/1 -> Mux3/9
  23/1 -> Mux3/8
  13/1 -> Mux3/7
  32/1 -> Mux3/6
  22/1 -> Mux3/5
  12/1 -> Mux3/4
  31/1 -> Mux3/3
  21/1 -> Mux3/2
  11/1 -> Mux3/1
  Reshape 9x1->3x3/1 -> Rw2b/1
  Mux3/1 -> Reshape 9x1->3x3/1

== system FixedWing_Dynamic_Model_SIL_simulink_PX4/Dynamics/Fixed-wing UAV Dynamics/Force and Moment Calculation/Aerodynamic Forces and Moments/Compute Body Frame Forces and Moments/Wind frame F& M/Lateral Channel/CY ==
  beta : Inport
  dR : Inport  Port=2
  CYDr : Constant  Value=uavData.aero.CYDr
      settings: AttributesFormatString=%<Value>
  CYb : Constant  Value=uavData.aero.CYb
      settings: AttributesFormatString=%<Value>
  Product : Product  SaturateOnIntegerOverflow=on  OutDataTypeStr=Inherit: Same as first input
  Product1 : Product  SaturateOnIntegerOverflow=on  OutDataTypeStr=Inherit: Same as first input
  Sum2 : Sum  SaturateOnIntegerOverflow=on
  CY : Outport  VectorParamsAs1DForOutWhenUnconnected=off
  wires:
  Product1/1 -> Sum2/2
  dR/1 -> Product1/2
  CYDr/1 -> Product1/1
  Product/1 -> Sum2/1
  Sum2/1 -> CY/1
  beta/1 -> Product/2
  CYb/1 -> Product/1

== system FixedWing_Dynamic_Model_SIL_simulink_PX4/Dynamics/Fixed-wing UAV Dynamics/Force and Moment Calculation/Aerodynamic Forces and Moments/Compute Body Frame Forces and Moments/Wind frame F& M/Lateral Channel/Cl ==
  beta : Inport
  dA : Inport  Port=2
  dR : Inport  Port=3
  p,q,r : Inport  Port=4
  Airspeed : Inport  Port=5
  ClDa : Constant  Value=uavData.aero.ClDa
      settings: AttributesFormatString=%<Value>
  ClDr : Constant  Value=uavData.aero.ClDr
      settings: AttributesFormatString=%<Value>
  Clb : Constant  Value=uavData.aero.Clb
      settings: AttributesFormatString=%<Value>
  Product1 : Product  SaturateOnIntegerOverflow=on  OutDataTypeStr=Inherit: Same as first input
  Product4 : Product  SaturateOnIntegerOverflow=on  OutDataTypeStr=Inherit: Same as first input
  Product5 : Product  SaturateOnIntegerOverflow=on  OutDataTypeStr=Inherit: Same as first input
  Sum : Sum  Inputs=+++++  SaturateOnIntegerOverflow=on
  roll factors : Subsystem
  Cl : Outport  VectorParamsAs1DForOutWhenUnconnected=off
  wires:
  roll factors/1(Clp) -> Sum/4
  Product5/1 -> Sum/2  "CldA"
  Airspeed/1 -> roll factors/2(Airspeed)
  p,q,r/1 -> roll factors/1(p,q,r)
  roll factors/2(Clr) -> Sum/5
  Product1/1 -> Sum/3  "Cldr"
  Product4/1 -> Sum/1  "Clb"
  Sum/1 -> Cl/1
  dR/1 -> Product1/2
  ClDr/1 -> Product1/1
  dA/1 -> Product5/2
  ClDa/1 -> Product5/1
  beta/1 -> Product4/2
  Clb/1 -> Product4/1

== system FixedWing_Dynamic_Model_SIL_simulink_PX4/Dynamics/Fixed-wing UAV Dynamics/Force and Moment Calculation/Aerodynamic Forces and Moments/Compute Body Frame Forces and Moments/Wind frame F& M/Lateral Channel/Cn ==
  beta : Inport
  dA : Inport  Port=2
  Dr : Inport  Port=3
  p,q,r : Inport  Port=4
  Airspeed : Inport  Port=5
  CnDa : Constant  Value=uavData.aero.CnDa
      settings: AttributesFormatString=%<Value>
  CnDr : Constant  Value=uavData.aero.CnDr
      settings: AttributesFormatString=%<Value>
  Cnb : Constant  Value=uavData.aero.Cnb
      settings: AttributesFormatString=%<Value>
  Product1 : Product  SaturateOnIntegerOverflow=on  OutDataTypeStr=Inherit: Same as first input
  Product4 : Product  SaturateOnIntegerOverflow=on  OutDataTypeStr=Inherit: Same as first input
  Product5 : Product  SaturateOnIntegerOverflow=on  OutDataTypeStr=Inherit: Same as first input
  Sum : Sum  Inputs=+++++  SaturateOnIntegerOverflow=on
  yaw factors : Subsystem
  Cn : Outport  VectorParamsAs1DForOutWhenUnconnected=off
  wires:
  Airspeed/1 -> yaw factors/2(Airspeed)
  p,q,r/1 -> yaw factors/1(p,q,r)
  Cnb/1 -> Product4/1
  beta/1 -> Product4/2
  CnDa/1 -> Product5/1
  Product5/1 -> Sum/2
  dA/1 -> Product5/2
  CnDr/1 -> Product1/1
  Dr/1 -> Product1/2
  Sum/1 -> Cn/1
  Product1/1 -> Sum/3
  yaw factors/2(Cnr) -> Sum/5
  yaw factors/1(Cnp) -> Sum/4
  Product4/1 -> Sum/1

== system FixedWing_Dynamic_Model_SIL_simulink_PX4/Dynamics/Fixed-wing UAV Dynamics/Force and Moment Calculation/Aerodynamic Forces and Moments/Compute Body Frame Forces and Moments/Wind frame F& M/Longitudinal Channel/CD ==
  CL : Inport
  Apolar : Constant  Value=uavData.aero.A1
      settings: AttributesFormatString=%<Value>
  Apolar (A2) : Constant  Value=uavData.aero.Apolar
      settings: AttributesFormatString=%<Value>
  CD0 : Constant  Value=uavData.aero.CD0
      settings: AttributesFormatString=%<Value>
  Gain : Gain  Gain=-1  SaturateOnIntegerOverflow=on  OutDataTypeStr=Inherit: Same as input  ParamDataTypeStr=Inherit: Same as input
      settings: AttributesFormatString=%<Gain>
  Math Function : Math  Operator=square  SignedPower=on
  Product : Product  SaturateOnIntegerOverflow=on  OutDataTypeStr=Inherit: Same as first input
  Product1 : Product  SaturateOnIntegerOverflow=on  OutDataTypeStr=Inherit: Same as first input
  Sum1 : Sum  Inputs=+++  SaturateOnIntegerOverflow=on
  CD : Outport  VectorParamsAs1DForOutWhenUnconnected=off
  wires:
  Gain/1 -> CD/1
  Apolar (A2)/1 -> Product/1
  Math Function/1 -> Product/2
  Product1/1 -> Sum1/3
  Product/1 -> Sum1/2
  CL/1 -> Math Function/1, Product1/1
  Sum1/1 -> Gain/1
  CD0/1 -> Sum1/1
  Apolar/1 -> Product1/2

== system FixedWing_Dynamic_Model_SIL_simulink_PX4/Dynamics/Fixed-wing UAV Dynamics/Force and Moment Calculation/Aerodynamic Forces and Moments/Compute Body Frame Forces and Moments/Wind frame F& M/Longitudinal Channel/CL ==
  alpha : Inport
  alpha_dot : Inport  Port=2
  dE : Inport  Port=3
  dF : Inport  Port=4
  p,q,r : Inport  Port=5
  Airspeed : Inport  Port=6
  CL0 : Constant  Value=uavData.aero.CL0
      settings: AttributesFormatString=%<Value>
  CLDe : Constant  Value=uavData.aero.CLDe
      settings: AttributesFormatString=%<Value>
  CLa : Constant  Value=uavData.aero.CLa
      settings: AttributesFormatString=%<Value>
  CLa_dot : Constant  Value=uavData.aero.CLa_dot
      settings: AttributesFormatString=%<Value>
  CmDe1 : Constant  Value=uavData.aero.CLDf
      settings: AttributesFormatString=%<Value>
  Lift due to pitch rate : Subsystem
  Product{1..2,4..5} (4 alike) : Product  SaturateOnIntegerOverflow=on  OutDataTypeStr=Inherit: Same as first input
  Sum : Sum  Inputs=++++++  SaturateOnIntegerOverflow=on
  CL : Outport  VectorParamsAs1DForOutWhenUnconnected=off
  wires:
  CL0/1 -> Sum/1
  Airspeed/1 -> Lift due to pitch rate/2(Airspeed)
  p,q,r/1 -> Lift due to pitch rate/1(p,q,r)
  Lift due to pitch rate/1(CLq) -> Sum/6
  Product2/1 -> Sum/5
  Product1/1 -> Sum/4
  Product5/1 -> Sum/3
  CmDe1/1 -> Product2/1
  dF/1 -> Product2/2
  Sum/1 -> CL/1
  dE/1 -> Product1/2
  CLDe/1 -> Product1/1
  alpha_dot/1 -> Product5/2
  CLa_dot/1 -> Product5/1
  alpha/1 -> Product4/2
  CLa/1 -> Product4/1
  Product4/1 -> Sum/2

== system FixedWing_Dynamic_Model_SIL_simulink_PX4/Dynamics/Fixed-wing UAV Dynamics/Force and Moment Calculation/Aerodynamic Forces and Moments/Compute Body Frame Forces and Moments/Wind frame F& M/Longitudinal Channel/Cm ==
  alpha : Inport
  De : Inport  Port=2
  Df : Inport  Port=3
  p,q,r : Inport  Port=4
  Cm0 : Constant  Value=uavData.aero.Cm0
      settings: AttributesFormatString=%<Value>
  CmDe : Constant  Value=uavData.aero.CmDe
      settings: AttributesFormatString=%<Value>
  CmDf : Constant  Value=uavData.aero.CmDf
      settings: AttributesFormatString=%<Value>
  Cma : Constant  Value=uavData.aero.Cma
      settings: AttributesFormatString=%<Value>
  Cma1 : Constant  Value=uavData.aero.Cmq
      settings: AttributesFormatString=%<Value>
  Get q : Selector  InputPortWidth=3  IndexOptions=Index vector (dialog)  Indices=2  OutputSizes=[(-2)]
  Product1 : Product  Inputs=***/  SaturateOnIntegerOverflow=on  OutDataTypeStr=Inherit: Same as first input
  Product2 : Product  SaturateOnIntegerOverflow=on  OutDataTypeStr=Inherit: Same as first input
  Product3 : Product  SaturateOnIntegerOverflow=on  OutDataTypeStr=Inherit: Same as first input
  Product4 : Product  SaturateOnIntegerOverflow=on  OutDataTypeStr=Inherit: Same as first input
  Sum : Sum  Inputs=+++++  SaturateOnIntegerOverflow=on
  chord : Constant  Value=uavData.geometry.chord
      settings: AttributesFormatString=%<Value>
  elarm : Constant  Value=uavData.geometry.elarm
      settings: AttributesFormatString=%<Value>
  Cm : Outport  VectorParamsAs1DForOutWhenUnconnected=off
  wires:
  chord/1 -> Product1/4
  elarm/1 -> Product1/3
  Get q/1 -> Product3/2
  Product3/1 -> Sum/5  "cmq"
  p,q,r/1 -> Get q/1
  Cma1/1 -> Product3/1
  Product1/1 -> Sum/3  "cmde"
  Product4/1 -> Sum/2  "cma"
  Sum/1 -> Cm/1  "total"
  De/1 -> Product1/2
  CmDe/1 -> Product1/1
  alpha/1 -> Product4/2
  Cma/1 -> Product4/1
  Df/1 -> Product2/2
  CmDf/1 -> Product2/1
  Product2/1 -> Sum/4  "cmdf"
  Cm0/1 -> Sum/1  "cm0"

== system FixedWing_Dynamic_Model_SIL_simulink_PX4/Dynamics/Fixed-wing UAV Dynamics/Force and Moment Calculation/Aerodynamic Forces and Moments/Compute Body Frame Forces and Moments/Wind frame F& M/Lateral Channel/Cl/roll factors ==
  p,q,r : Inport
  Airspeed : Inport  Port=2
  Constant : Constant  Value=uavData.aero.Clp
      settings: AttributesFormatString=%<Value>
  Constant1 : Constant  Value=uavData.aero.Clr
      settings: AttributesFormatString=%<Value>
  Get p : Selector  InputPortWidth=3  IndexOptions=Index vector (dialog)  Indices=1  OutputSizes=[(-2)]
  Get r : Selector  InputPortWidth=3  IndexOptions=Index vector (dialog)  Indices=3  OutputSizes=[(-2)]
  Product : Product  SaturateOnIntegerOverflow=on  OutDataTypeStr=Inherit: Same as first input
  Product1 : Product  SaturateOnIntegerOverflow=on  OutDataTypeStr=Inherit: Same as first input
  roll rate fact : Subsystem
  yaw rate fact : Subsystem
  Clp : Outport  VectorParamsAs1DForOutWhenUnconnected=off
  Clr : Outport  Port=2  VectorParamsAs1DForOutWhenUnconnected=off
  wires:
  Get r/1 -> yaw rate fact/1(r)
  p,q,r/1 -> Get r/1, Get p/1
  Get p/1 -> roll rate fact/1(p)
  Airspeed/1 -> yaw rate fact/2(Airspeed), roll rate fact/2(Airspeed)
  yaw rate fact/1(Yaw Rate Fac) -> Product1/2
  Constant1/1 -> Product1/1
  roll rate fact/1(Roll Rate Fac) -> Product/2
  Constant/1 -> Product/1
  Product1/1 -> Clr/1
  Product/1 -> Clp/1

== system FixedWing_Dynamic_Model_SIL_simulink_PX4/Dynamics/Fixed-wing UAV Dynamics/Force and Moment Calculation/Aerodynamic Forces and Moments/Compute Body Frame Forces and Moments/Wind frame F& M/Lateral Channel/Cn/yaw factors ==
  p,q,r : Inport
  Airspeed : Inport  Port=2
  Constant : Constant  Value=uavData.aero.Cnp
      settings: AttributesFormatString=%<Value>
  Constant1 : Constant  Value=uavData.aero.Cnr
      settings: AttributesFormatString=%<Value>
  Get p : Selector  InputPortWidth=3  IndexOptions=Index vector (dialog)  Indices=1  OutputSizes=[(-2)]
  Get r : Selector  InputPortWidth=3  IndexOptions=Index vector (dialog)  Indices=3  OutputSizes=[(-2)]
  Product : Product  SaturateOnIntegerOverflow=on  OutDataTypeStr=Inherit: Same as first input
  Product1 : Product  SaturateOnIntegerOverflow=on  OutDataTypeStr=Inherit: Same as first input
  roll rate fact : Subsystem
  yaw rate fact : Subsystem
  Cnp : Outport  VectorParamsAs1DForOutWhenUnconnected=off
  Cnr : Outport  Port=2  VectorParamsAs1DForOutWhenUnconnected=off
  wires:
  Airspeed/1 -> yaw rate fact/2(Airspeed), roll rate fact/2(Airspeed)
  Get r/1 -> yaw rate fact/1(r)
  p,q,r/1 -> Get r/1, Get p/1
  Get p/1 -> roll rate fact/1(p)
  roll rate fact/1(Roll Rate Fac) -> Product/2
  Constant/1 -> Product/1
  yaw rate fact/1(Yaw Rate Fac) -> Product1/2
  Constant1/1 -> Product1/1
  Product1/1 -> Cnr/1
  Product/1 -> Cnp/1

== system FixedWing_Dynamic_Model_SIL_simulink_PX4/Dynamics/Fixed-wing UAV Dynamics/Force and Moment Calculation/Aerodynamic Forces and Moments/Compute Body Frame Forces and Moments/Wind frame F& M/Longitudinal Channel/CL/Lift due to pitch rate ==
  p,q,r : Inport
  Airspeed : Inport  Port=2
  Constant : Constant  Value=uavData.aero.CLq
      settings: AttributesFormatString=%<Value>
  Get q : Selector  InputPortWidth=3  IndexOptions=Index vector (dialog)  Indices=2  OutputSizes=[(-2)]
  Product : Product  SaturateOnIntegerOverflow=on  OutDataTypeStr=Inherit: Same as first input
  pitch rate factor : Subsystem
  CLq : Outport  VectorParamsAs1DForOutWhenUnconnected=off
  wires:
  Airspeed/1 -> pitch rate factor/2(Airspeed)
  Get q/1 -> pitch rate factor/1(q)
  p,q,r/1 -> Get q/1
  Product/1 -> CLq/1
  pitch rate factor/1(Pitch Rate Fac) -> Product/2
  Constant/1 -> Product/1
